simulink model "wahdlo_model2"  (R2016a)
settings: Solver=ode4  StartTime=0.0  StopTime=15  FixedStep=0.001  RelTol=1e-3
values from neighbouring files (symbols this model uses):
  c1 = 5.8    [Epsilon.m]
  c2 = -18    [Epsilon.m]
  D = zeros(4,1)    [Epsilon.m]
  g = 9.81    [Epsilon.m]
  Jr = J_sm + m_wah*L^2    [Epsilon.m]
  L = srodek_ciez-d_wystajacego    (= 0.252)    [init2.m]    (also in params.mat)
  M = 0.530    (= 0.53)    [Epsilon.m]
  m_wah = 2*(m_ciezarka + m_rurki)    (= 0.062)    [init2.m]    (also in params.mat)
undefined symbols (not defined in the file or in its folder): sigbuilder_block
settings Model: Creator=Mike  LastModifiedBy=Mike

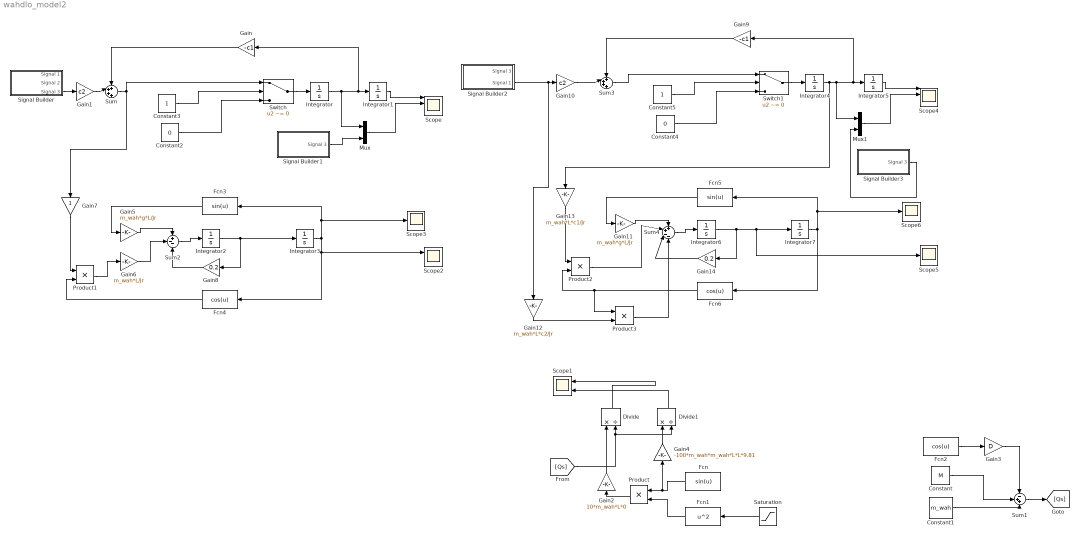
== system wahdlo_model2 ==
  Constant : Constant  Value=M
  Constant1 : Constant  Value=m_wah
  Constant2 : Constant  Value=0
  Constant3 : Constant
  Constant4 : Constant  Value=0
  Constant5 : Constant
  Divide : Product  Inputs=*/
  Divide1 : Product  Inputs=*/
  Fcn : Fcn  Expr=sin(u)
  Fcn1 : Fcn  Expr=u^2
  Fcn2 : Fcn  Expr=cos(u)
  Fcn3 : Fcn  Expr=sin(u)
  Fcn4 : Fcn  Expr=cos(u)
  Fcn5 : Fcn  Expr=sin(u)
  Fcn6 : Fcn  Expr=cos(u)
  Gain : Gain  Gain=-c1
  Gain1 : Gain  Gain=c2
  Gain10 : Gain  Gain=c2
  Gain11 : Gain  Gain=m_wah*g*L/Jr
  Gain12 : Gain  Gain=m_wah*L*c2/Jr
  Gain13 : Gain  Gain=m_wah*L*c1/Jr
  Gain14 : Gain  Gain=0.2
  Gain2 : Gain  Gain=10*m_wah*L*0
  Gain3 : Gain  Gain=D
  Gain4 : Gain  Gain=-100*m_wah*m_wah*L*L*9.81
  Gain5 : Gain  Gain=m_wah*g*L/Jr
  Gain6 : Gain  Gain=m_wah*L/Jr
  Gain7 : Gain
  Gain8 : Gain  Gain=0.2
  Gain9 : Gain  Gain=-c1
  Integrator{,1..2,4..6} (6 alike) : Integrator
  Integrator3 : Integrator  InitialCondition=pi
  Integrator7 : Integrator  InitialCondition=pi
  Mux : Mux  Inputs=2
  Mux1 : Mux  Inputs=2
  Product{,1..3} (4 alike) : Product
  Saturation : Saturate  UpperLimit=10  LowerLimit=-10
  Scope : Scope  NumInputPorts=4
  Scope1 : Scope  NumInputPorts=2
  Scope2 : Scope  NumInputPorts=2
  Scope3 : Scope
  Scope4 : Scope  NumInputPorts=4
  Scope5 : Scope
  Scope6 : Scope
  Signal Builder : Subsystem  Tag=STV Subsys  LoadFcn=sigbuilder_block('load');  StartFcn=sigbuilder_block('start');  StopFcn=sigbuilder_block('stop');  ClipboardFcn=sigbuilder_block('clipboard');  mask(Sigbuilder block){}
      mask help: Simulink:masks:SigbuilderBlock_MD
      mask init:
      | if ~strcmp(get_param(bdroot(gcbh),'SimulationStatus'),'stopped') tuvar = sigbuilder_block('maskInit'); end
      settings: CopyFcn=sigbuilder_block('copy');  DeleteFcn=sigbuilder_block('delete');  ModelCloseFcn=sigbuilder_block('modelClose');  PreSaveFcn=sigbuilder_block('preSave');  PauseFcn=sigbuilder_block('pause');  ContinueFcn=sigbuilder_block('continue');  NameChangeFcn=sigbuilder_block('namechange');  OpenFcn=sigbuilder_block('open',[437.6 199.2 550.4 400 ]);  CloseFcn=sigbuilder_block('close');
      mask Display: plot(0, 0, 100, 100,[2, 2, 32, 32, 2], [68, 8, 8, 68, 68],[32, 2], [38, 38], [32, 19, 2],[53, 60, 44], [32, 17, 17, 2],[16, 16, 31, 31]);txt = getActiveGroup(gcbh);text(2, 100, txt,'verticalAlignment', 'top');
  Signal Builder1 : Subsystem  Tag=STV Subsys  LoadFcn=sigbuilder_block('load');  StartFcn=sigbuilder_block('start');  StopFcn=sigbuilder_block('stop');  ClipboardFcn=sigbuilder_block('clipboard');  mask(Sigbuilder block){}
      mask help: Simulink:masks:SigbuilderBlock_MD
      mask init:
      | if ~strcmp(get_param(bdroot(gcbh),'SimulationStatus'),'stopped') tuvar = sigbuilder_block('maskInit'); end
      settings: CopyFcn=sigbuilder_block('copy');  DeleteFcn=sigbuilder_block('delete');  ModelCloseFcn=sigbuilder_block('modelClose');  PreSaveFcn=sigbuilder_block('preSave');  PauseFcn=sigbuilder_block('pause');  ContinueFcn=sigbuilder_block('continue');  NameChangeFcn=sigbuilder_block('namechange');  OpenFcn=sigbuilder_block('open',[437.6 199.2 550.4 400 ]);  CloseFcn=sigbuilder_block('close');
      mask Display: plot(0, 0, 100, 100,[2, 2, 32, 32, 2], [68, 8, 8, 68, 68],[32, 2], [38, 38], [32, 19, 2],[53, 60, 44], [32, 17, 17, 2],[16, 16, 31, 31]);txt = getActiveGroup(gcbh);text(2, 100, txt,'verticalAlignment', 'top');
  Signal Builder2 : Subsystem  Tag=STV Subsys  LoadFcn=sigbuilder_block('load');  StartFcn=sigbuilder_block('start');  StopFcn=sigbuilder_block('stop');  ClipboardFcn=sigbuilder_block('clipboard');  mask(Sigbuilder block){}
      mask help: Simulink:masks:SigbuilderBlock_MD
      mask init:
      | if ~strcmp(get_param(bdroot(gcbh),'SimulationStatus'),'stopped') tuvar = sigbuilder_block('maskInit'); end
      settings: CopyFcn=sigbuilder_block('copy');  DeleteFcn=sigbuilder_block('delete');  ModelCloseFcn=sigbuilder_block('modelClose');  PreSaveFcn=sigbuilder_block('preSave');  PauseFcn=sigbuilder_block('pause');  ContinueFcn=sigbuilder_block('continue');  NameChangeFcn=sigbuilder_block('namechange');  OpenFcn=sigbuilder_block('open',[6 0 1428 711.75 ]);  CloseFcn=sigbuilder_block('close');
      mask Display: plot(0, 0, 100, 100,[2, 2, 32, 32, 2], [68, 8, 8, 68, 68],[32, 2], [38, 38], [32, 19, 2],[53, 60, 44], [32, 17, 17, 2],[16, 16, 31, 31]);txt = getActiveGroup(gcbh);text(2, 100, txt,'verticalAlignment', 'top');
  Signal Builder3 : Subsystem  Tag=STV Subsys  LoadFcn=sigbuilder_block('load');  StartFcn=sigbuilder_block('start');  StopFcn=sigbuilder_block('stop');  ClipboardFcn=sigbuilder_block('clipboard');  mask(Sigbuilder block){}
      mask help: Simulink:masks:SigbuilderBlock_MD
      mask init:
      | if ~strcmp(get_param(bdroot(gcbh),'SimulationStatus'),'stopped') tuvar = sigbuilder_block('maskInit'); end
      settings: CopyFcn=sigbuilder_block('copy');  DeleteFcn=sigbuilder_block('delete');  ModelCloseFcn=sigbuilder_block('modelClose');  PreSaveFcn=sigbuilder_block('preSave');  PauseFcn=sigbuilder_block('pause');  ContinueFcn=sigbuilder_block('continue');  NameChangeFcn=sigbuilder_block('namechange');  OpenFcn=sigbuilder_block('open',[437.6 199.2 550.4 400 ]);  CloseFcn=sigbuilder_block('close');
      mask Display: plot(0, 0, 100, 100,[2, 2, 32, 32, 2], [68, 8, 8, 68, 68],[32, 2], [38, 38], [32, 19, 2],[53, 60, 44], [32, 17, 17, 2],[16, 16, 31, 31]);txt = getActiveGroup(gcbh);text(2, 100, txt,'verticalAlignment', 'top');
  Sum : Sum  Inputs=4
  Sum1 : Sum  Inputs=-++
  Sum2 : Sum  Inputs=+--
  Sum3 : Sum  Inputs=4
  Sum4 : Sum  Inputs=++--
  Switch : Switch  Criteria=u2 ~= 0
  Switch1 : Switch  Criteria=u2 ~= 0
  wires:
  Integrator/1 -> Mux/1, Gain/1, Integrator1/1
  Sum/1 -> Switch/1, Gain7/1
  Gain/1 -> Sum/1
  Gain1/1 -> Sum/2
  Signal Builder1/1(Signal 3) -> Mux/2
  ? -> Fcn2/1, Fcn/1
  ? -> Saturation/1
  Fcn/1 -> Gain4/1, Product/1
  Fcn1/1 -> Product/2
  Constant/1 -> Sum1/2
  Constant1/1 -> Sum1/3
  Fcn2/1 -> Gain3/1
  Gain3/1 -> Sum1/1
  [Qs] -> Divide1/2, Divide/2
  Gain2/1 -> Divide/1
  Product/1 -> Gain2/1
  Divide/1 -> Scope1/1
  Gain4/1 -> Divide1/1
  Divide1/1 -> Scope1/2
  Sum1/1 -> [Qs]
  Integrator1/1 -> Scope/1
  Mux/1 -> Scope/2
  Saturation/1 -> Fcn1/1
  Integrator2/1 -> Gain8/1, Integrator3/1
  Gain5/1 -> Sum2/1
  Integrator3/1 -> Scope2/1, Fcn4/1, Scope3/1, Fcn3/1
  Fcn3/1 -> Gain5/1
  Fcn4/1 -> Product1/2
  Product1/1 -> Gain6/1
  Gain6/1 -> Sum2/2
  Gain7/1 -> Product1/1
  Signal Builder/3(Signal 3) -> Gain1/1
  Gain8/1 -> Sum2/3
  Sum2/1 -> Integrator2/1
  Switch/1 -> Integrator/1
  Constant2/1 -> Switch/3
  Constant3/1 -> Switch/2
  Integrator4/1 -> Gain13/1, Mux1/1, Gain9/1, Integrator5/1
  Sum3/1 -> Switch1/1
  Gain9/1 -> Sum3/1
  Gain10/1 -> Sum3/2
  Signal Builder3/1(Signal 3) -> Mux1/2
  Integrator5/1 -> Scope4/1
  Mux1/1 -> Scope4/2
  Integrator6/1 -> Gain14/1, Scope5/1, Integrator7/1
  Gain11/1 -> Sum4/1
  Integrator7/1 -> Fcn6/1, Scope6/1, Fcn5/1
  Fcn5/1 -> Gain11/1
  Fcn6/1 -> Product3/1, Product2/2
  Product2/1 -> Sum4/2
  Gain13/1 -> Product2/1
  Signal Builder2/2(Signal 1) -> Gain12/1, Gain10/1
  Gain14/1 -> Sum4/3
  Sum4/1 -> Integrator6/1
  Switch1/1 -> Integrator4/1
  Constant4/1 -> Switch1/3
  Constant5/1 -> Switch1/2
  Gain12/1 -> Product3/2
  Product3/1 -> Sum4/4

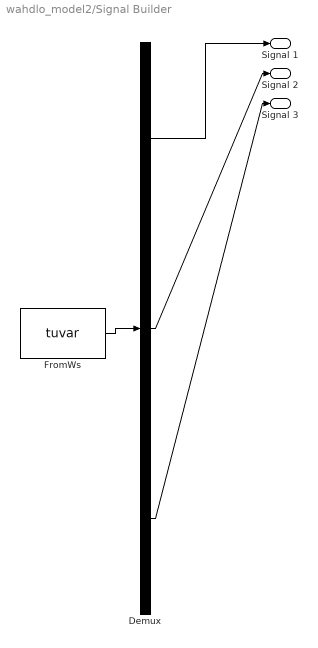
== system wahdlo_model2/Signal Builder ==
  Demux : Demux  Tag=STV Demux  Outputs=3
  FromWs : FromWorkspace  Tag=STV FromWs  VariableName=tuvar  SampleTime=0
      SigBuilderData=|
      | common.afterFinalStr = 'Extrapolate'
      | common.sampleTime = 0
      | dataSet.timeRange = [0 30]
      | dataSet.name = 'Group 1'
      | sbobj.Groups.Name = 'Group 1'
      | sbobj.Groups.Signals(1).Name = 'Signal 1'
      | sbobj.Groups.Signals(1).XData = [0 4 4 6 6 30]
      | sbobj.Groups.Signals(1).YData = [0 0 0.28 0.28 0 0]
      | sbobj.Groups.Signals(2).Name = 'Signal 2'
      | sbobj.Groups.Signals(2).XData = [0 0.01 0.02 0.03 0.04 0.05 0.06 0.07 0.08 0.09 0.1 0.11 ... (1001 elements, 1x1001)]
      | sbobj.Groups.Signals(2).YData = [0.1 0.1 0.1 0.1 0.1 0.1 0.1 0.1 0.1 0.1 0.1 0.1 ... (1001 elements, 1x1001)]
      | sbobj.Groups.Signals(3).Name = 'Signal 3'
      | sbobj.Groups.Signals(3).XData = [0 0.01 0.02 0.03 0.04 0.05 0.06 0.07 0.08 0.09 0.1 0.11 ... (3001 elements, 1x3001)]
      | sbobj.Groups.Signals(3).YData = [0.1 0.1 0.1 0.1 0.1 0.1 0.1 0.1 0.1 0.1 0.1 0.1 ... (3001 elements, 1x3001)]
      | sbobj.Groups.TimeRange = [0 30]
  Signal 1 : Outport  Tag=STV Outport
  Signal 2 : Outport  Tag=STV Outport  Port=2
  Signal 3 : Outport  Tag=STV Outport  Port=3
  wires:
  Demux/1 -> Signal 1/1
  FromWs/1 -> Demux/1
  Demux/2 -> Signal 2/1
  Demux/3 -> Signal 3/1

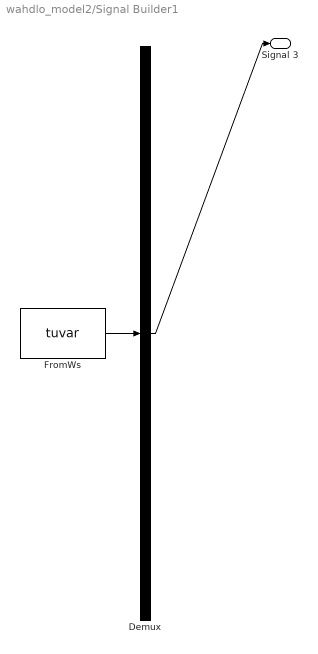
== system wahdlo_model2/Signal Builder1 ==
  Demux : Demux  Tag=STV Demux  Outputs=1
  FromWs : FromWorkspace  Tag=STV FromWs  VariableName=tuvar  SampleTime=0
      SigBuilderData=|
      | common.afterFinalStr = 'Extrapolate'
      | common.sampleTime = 0
      | dataSet.timeRange = [0 30]
      | dataSet.name = 'Group 1'
      | sbobj.Groups.Name = 'Group 1'
      | sbobj.Groups.Signals.Name = 'Signal 3'
      | sbobj.Groups.Signals.XData = [0 0.01 0.02 0.03 0.04 0.05 0.06 0.07 0.08 0.09 0.1 0.11 ... (3001 elements, 1x3001)]
      | sbobj.Groups.Signals.YData = [2.0902351 0 -0.0057053 -0.0114106 -0.0171159 -0.0171159 -0.0171159 -0.0171159 -0.0171159 -0.0114106 -0.0114106 -0.0114106 ... (3001 elements, 1x3001)]
      | sbobj.Groups.TimeRange = [0 30]
  Signal 3 : Outport  Tag=STV Outport
  wires:
  FromWs/1 -> Demux/1
  Demux/1 -> Signal 3/1

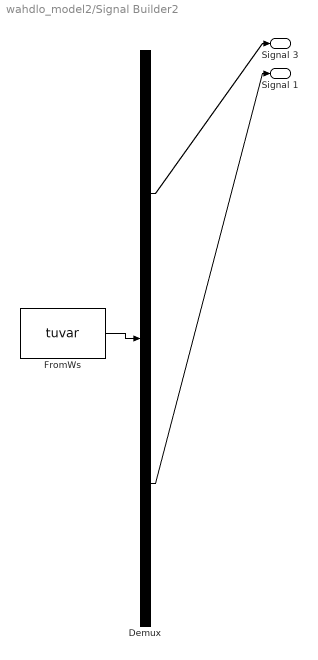
== system wahdlo_model2/Signal Builder2 ==
  Demux : Demux  Tag=STV Demux  Outputs=2
  FromWs : FromWorkspace  Tag=STV FromWs  VariableName=tuvar  SampleTime=0
      SigBuilderData=|
      | common.afterFinalStr = 'Extrapolate'
      | common.sampleTime = 0
      | dataSet.timeRange = [0 30]
      | dataSet.name = 'Group 1'
      | sbobj.Groups.Name = 'Group 1'
      | sbobj.Groups.Signals(1).Name = 'Signal 3'
      | sbobj.Groups.Signals(1).XData = [0 0.01 0.02 0.03 0.04 0.05 0.06 0.07 0.08 0.09 0.1 0.11 ... (3001 elements, 1x3001)]
      | sbobj.Groups.Signals(1).YData = [0.1 0.1 0.1 0.1 0.1 0.1 0.1 0.1 0.1 0.1 0.1 0.1 ... (3001 elements, 1x3001)]
      | sbobj.Groups.Signals(2).Name = 'Signal 1'
      | sbobj.Groups.Signals(2).XData = [0 0.01 0.02 0.03 0.04 0.05 0.06 0.07 0.08 0.09 0.1 0.11 ... (3001 elements, 1x3001)]
      | sbobj.Groups.Signals(2).YData = [0 0 0 0 0 0 0 0 0 0 0 0 ... (3001 elements, 1x3001)]
      | sbobj.Groups.TimeRange = [0 30]
  Signal 3 : Outport  Tag=STV Outport
  Signal 1 : Outport  Tag=STV Outport  Port=2
  wires:
  FromWs/1 -> Demux/1
  Demux/1 -> Signal 3/1
  Demux/2 -> Signal 1/1

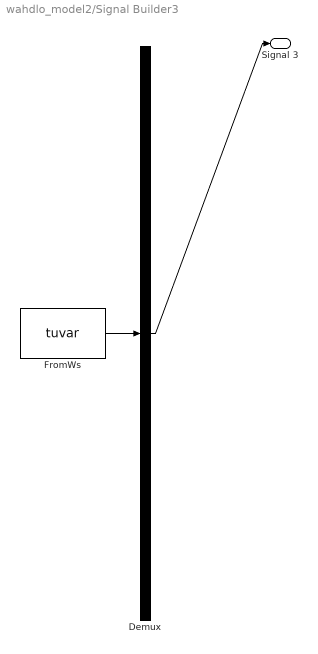
== system wahdlo_model2/Signal Builder3 ==
  Demux : Demux  Tag=STV Demux  Outputs=1
  FromWs : FromWorkspace  Tag=STV FromWs  VariableName=tuvar  SampleTime=0
      SigBuilderData=|
      | common.afterFinalStr = 'Extrapolate'
      | common.sampleTime = 0
      | dataSet.timeRange = [0 30]
      | dataSet.name = 'Group 1'
      | sbobj.Groups.Name = 'Group 1'
      | sbobj.Groups.Signals.Name = 'Signal 3'
      | sbobj.Groups.Signals.XData = [0 0.01 0.02 0.03 0.04 0.05 0.06 0.07 0.08 0.09 0.1 0.11 ... (3001 elements, 1x3001)]
      | sbobj.Groups.Signals.YData = [2.0902351 0 -0.0057053 -0.0114106 -0.0171159 -0.0171159 -0.0171159 -0.0171159 -0.0171159 -0.0114106 -0.0114106 -0.0114106 ... (3001 elements, 1x3001)]
      | sbobj.Groups.TimeRange = [0 30]
  Signal 3 : Outport  Tag=STV Outport
  wires:
  FromWs/1 -> Demux/1
  Demux/1 -> Signal 3/1
